simulink model "Statechart_Test_3"  (R2016b)
settings: Solver=VariableStepAuto  StartTime=0.0  StopTime=10.0  RelTol=1e-3  EnableMultiTasking=on
settings Model: Creator=Rose  LastModifiedBy=Rose
settings OptimizationCC: DefaultParameterBehavior=Inlined  LifeSpan=inf
settings DebuggingCC: SFUnexpectedBacktrackingDiag=warning  SFNoUnconditionalDefaultTransitionDiag=warning  SFExecutionAtInitializationDiag=none
settings GRTTargetCC: TargetLangStandard=C89/C90 (ANSI)
settings ConfigComp: CovMetricSettings=dw  CovHtmlReporting=on  CovSaveCumulativeToWorkspaceVar=on  CovSaveSingleToWorkspaceVar=on  CovExternalEMLEnable=off

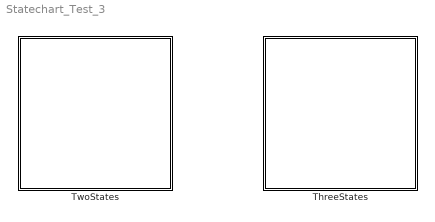
== system Statechart_Test_3 ==
  ThreeStates : Stateflow chart  TreatAsAtomicUnit=on
  TwoStates : Stateflow chart  TreatAsAtomicUnit=on

== stateflow chart Statechart_Test_3/ThreeStates ==
  state InitializeSystem
  state On
  state FailState
  (default) -> InitializeSystem
  FailState -> InitializeSystem
  InitializeSystem -> On [order 1]
  InitializeSystem -> FailState [order 2]
  On -> FailState

== stateflow chart Statechart_Test_3/TwoStates ==
  state ON
  state OFF
  (default) -> ON
  OFF -> ON
  ON -> OFF
